simulink library "INT_CoVM_TrqLeadCoord"  (R2016b)
settings: Solver=VariableStepAuto  StartTime=0.0  StopTime=10.0  RelTol=1e-3
settings Model: Creator=bianxuyin  LastModifiedBy=bianxuyin

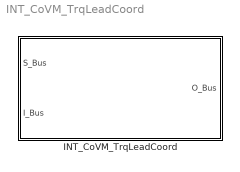
== system INT_CoVM_TrqLeadCoord ==
  INT_CoVM_TrqLeadCoord : Subsystem

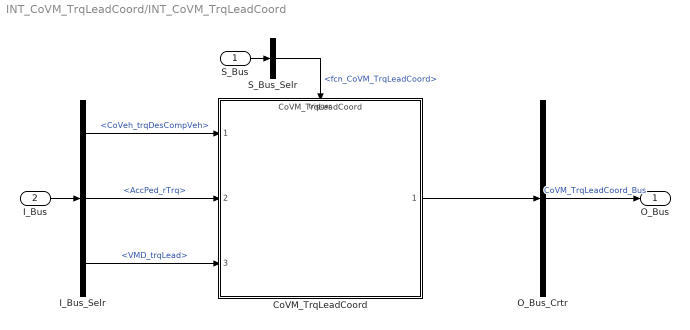
== system INT_CoVM_TrqLeadCoord/INT_CoVM_TrqLeadCoord ==
  S_Bus : Inport
  I_Bus : Inport  Port=2
  CoVM_TrqLeadCoord : ModelReference  ModelNameDialog=CoVM_TrqLeadCoord  SimulationMode=Normal  ModelReferenceVersion=1.4  TriggerPortName=function  TriggerPortTriggerType=function-call  TriggerPortStatesWhenEnabling=held
  I_Bus_Selr : BusSelector  OutputSignals=CoVeh_trqDesCompVeh,AccPed_rTrq,VMD_trqLead
  O_Bus_Crtr : BusCreator  Inputs=1
  S_Bus_Selr : BusSelector  OutputSignals=fcn_CoVM_TrqLeadCoord
  O_Bus : Outport
  wires:
  S_Bus_Selr/1 -> CoVM_TrqLeadCoord/Trigger  "<fcn_CoVM_TrqLeadCoord>"
  S_Bus/1 -> S_Bus_Selr/1
  I_Bus/1 -> I_Bus_Selr/1
  I_Bus_Selr/1 -> CoVM_TrqLeadCoord/1  "<CoVeh_trqDesCompVeh>"
  I_Bus_Selr/2 -> CoVM_TrqLeadCoord/2  "<AccPed_rTrq>"
  I_Bus_Selr/3 -> CoVM_TrqLeadCoord/3  "<VMD_trqLead>"
  O_Bus_Crtr/1 -> O_Bus/1  "CoVM_TrqLeadCoord_Bus"
  CoVM_TrqLeadCoord/1 -> O_Bus_Crtr/1
